simulink model "rev0BB"  (R2017b)
settings: Solver=FixedStepDiscrete  StartTime=0  StopTime=(((preLen+100+dataLenSymbols)*1+pad_first*3)*basePer)  RelTol=1e-3
values from neighbouring files (symbols this model uses):
  ack_stf_len_symbols = length(x_ACK_STF)    [rev0BB_setup.m]
  agc_delay_lag = 32    [rev0BB_setup.m]
  agc_detector_coef = ones(1,agc_detector_taps)./agc_detector_taps    [rev0BB_setup.m]
  agc_on = true    [rev0BB_startup.m]
  agc_sat_low = -agcSaturation    (= -12)    [rev0BB_setup.m]
  agc_sat_up = agcSaturation    (= 12)    [rev0BB_setup.m]
  agcDesired = 0    [rev0BB_setup.m]
  agcExpDomain = agcSaturation    (= 12)    [rev0BB_setup.m]
  agcExpResolution = 2^-5    (= 0.03125)    [rev0BB_setup.m]
  agcPwrAvgNum = 128    [rev0BB_setup.m]
  agcSaturation = 12    [rev0BB_setup.m]
  agcSettleThresh = 0.65    [rev0BB_setup.m]
  agcStep = 2^-8    (= 0.00390625)    [rev0BB_setup.m]
  atanDomain = 5    [rev0BB_setup.m]
  atanDomainTiming = 256    [rev0BB_setup.m]
  atanResolution = 2^-9    (= 0.001953125)    [rev0BB_setup.m]
  atanResolutionTiming = 2^-5    (= 0.03125)    [rev0BB_setup.m]
  averaging_num = ones(1, averaging_samples)    [rev0BB_setup.m]
  averaging_samples = 128    [rev0BB_setup.m]
  awgnSeed = abs(dBSnrRange(dBSnrInd)*1000+trial+10000000)    [plotBer.m]    (also in rev0BB_startup.m = 67)
  basePer = 1/baseFreq    (= 5e-08)    [rev0BB_setup.m]
  bitsPerSymbolHeader = log2(radixHeader)    [rev0BB_setup.m]
  bitsPerSymbolMax = log2(radixMax)    [rev0BB_setup.m]
  cal_sig_i_mult = 1.0    (= 1)    [rev0BB_startup.m]
  cal_sig_i_offset = 0.0    (= 0)    [rev0BB_startup.m]
  cal_sig_q_mult = 1.0    (= 1)    [rev0BB_startup.m]
  cal_sig_q_offset = 0.0    (= 0)    [rev0BB_startup.m]
  cefEarlyWarning = 256    [rev0BB_setup.m]
  cefLen = length(x_CEF)    [rev0BB_setup.m]
  channelFIR = zeros(1, round(maxSampleDelay)+1)    [rev0BB_startup.m]
  coarseCFOAdaptDelay = 1    [rev0BB_setup.m]
  cr_i = 0.020    (= 0.02)    [rev0BB_setup.m]
  cr_i_preamp = 2^-9    (= 0.001953125)    [rev0BB_setup.m]
  cr_int1_sat_low = -cr_integrator1_saturation    (= -0.6)    [rev0BB_setup.m]
  cr_int1_sat_up = cr_integrator1_saturation    (= 0.6)    [rev0BB_setup.m]
  cr_integrator1_decay = 1    [rev0BB_setup.m]
  cr_integrator1_saturation = 0.6    [rev0BB_setup.m]
  cr_mult_pipeline = 0    [rev0BB_setup.m]
  cr_p = 0.015    [rev0BB_setup.m]
  cr_sat2_low = -cr_saturation2    (= -0.6)    [rev0BB_setup.m]
  cr_sat2_up = cr_saturation2    (= 0.6)    [rev0BB_setup.m]
  cr_smooth_num = (1/cr_smooth_samples).*ones(1, cr_smooth_samples)    [rev0BB_setup.m]
  D_128 = [ 1,  8,  2,  4, 16, 32, 64]    [golay.m]    (also in rev0BB_setup.m)
  D_32 = [ 1,  4,  8,  2, 16]    [golay.m]    (also in rev0BB_setup.m)
  dataLenSymbols = header_len_bytes*8/bitsPerSymbolHeader + frame_len_bytes*8/bitsPerSymbol    [rev0BB_setup.m]
  default_channel = 3    [rev0BB_setup.m]
  dmm_coefs = ones(1,dmm_samples)./dmm_samples    [rev0BB_setup.m]
  dst_field_len = 8    [rev0BB_setup.m]
  expDomain = 3.3    [rev0BB_setup.m]
  expResolution = 2^-5    (= 0.03125)    [rev0BB_setup.m]
  expTol = .1    (= 0.1)    [rev0BB_setup.m]
  flush_delay = regular_pipeline*2+mult_pipeline+4    (= 4)    [rev0BB_setup.m]
  frac_lut_domain = 256    [rev0BB_setup.m]
  frac_lut_domain_cr = 64    [rev0BB_setup.m]
  frac_lut_range_max = 512    [rev0BB_setup.m]
  frac_lut_range_max_coarse_cfo = 127    [rev0BB_setup.m]
  frac_lut_range_max_cr = 127    [rev0BB_setup.m]
  frac_lut_range_min = -frac_lut_range_max    (= -512)    [rev0BB_setup.m]
  frac_lut_range_min_coarse_cfo = -frac_lut_range_max_coarse_cfo    (= -127)    [rev0BB_setup.m]
  frac_lut_range_min_cr = -frac_lut_range_max_cr    (= -127)    [rev0BB_setup.m]
  frac_lut_table_breaks = -frac_lut_domain:frac_lut_res:(frac_lut_domain-1)    [rev0BB_setup.m]
  frac_lut_table_breaks_coarse_cfo = -frac_lut_domain_coarse_cfo:frac_lut_res_coarse_cfo:(frac_lut_domain_coarse_cfo-1)    [rev0BB_setup.m]
  frac_lut_table_breaks_cr = -frac_lut_domain_cr:frac_lut_res_cr:(frac_lut_domain_cr-1)    [rev0BB_setup.m]
  frac_lut_table_data = 1./frac_lut_table_breaks    [rev0BB_setup.m]
  frac_lut_table_data_coarse_cfo = 1./frac_lut_table_breaks_coarse_cfo    [rev0BB_setup.m]
  frac_lut_table_data_cr = 1./frac_lut_table_breaks_cr    [rev0BB_setup.m]
  freeze_en_agc = true    [rev0BB_startup.m]
  freeze_en_cr_int1 = false    [rev0BB_startup.m]
  freeze_en_cr_int2 = false    [rev0BB_startup.m]
  freeze_en_cr_phase = false    [rev0BB_startup.m]
  freeze_en_tr_int1 = false    [rev0BB_startup.m]
  freeze_en_tr_int2 = false    [rev0BB_startup.m]
  freeze_en_tr_phase = false    [rev0BB_startup.m]
  freeze_on_cef_done = true    [rev0BB_startup.m]
  freeze_on_stf_done = false    [rev0BB_startup.m]
  freeze_on_valid = true    [rev0BB_startup.m]
  golay_type = 32    [rev0BB_setup.m]
  guardInt = int16(4)    [rev0BB_setup.m]
  guardTol = int16(5)    [rev0BB_setup.m]
  header_len_bytes = 8    [rev0BB_setup.m]
  lineWidth = 60    [rev0BB_setup.m]
  lmsEqDepth = 38    [rev0BB_setup.m]
  lmsStep_init = 0.006    [rev0BB_setup.m]
  lmsStep_meta = (lmsStep_final - lmsStep_init)/cefLen    [rev0BB_setup.m]
  lnDomain = 16    [rev0BB_setup.m]
  lnResolution = 2^-5    (= 0.03125)    [rev0BB_setup.m]
  local_node_id = 2    [rev0BB_startup.m]
  maxMsgSize = length(xSpectrum_PRE)+dataLenSymbols+300    [rev0BB_setup.m]
  minSTFPeaks = 3    [rev0BB_setup.m]
  mod_scheme_len_bytes = 1    [rev0BB_setup.m]
  modBPS = [1, 2, 4]    [rev0BB_setup.m]
  modKeys = [0, 1, 2]    [rev0BB_setup.m]
  mult_pipeline = 0    [rev0BB_setup.m]
  overSampleFreq = 80e6    (= 80000000)    [rev0BB_setup.m]
  overSamplePer = 1/overSampleFreq    (= 1.25e-08)    [rev0BB_setup.m]
  pad_first = 1000    [createTestVectors.m]
  post_cr_i_offset = 0    [rev0BB_startup.m]
  post_cr_q_offset = 0    [rev0BB_startup.m]
  preambleSequentialDetect = 2    [rev0BB_setup.m]
  preLen = length(x_PRE)    [rev0BB_setup.m]
  qam16_demod_scale_factor = qam16_hdl_distance/qam16_power_normalized_distance    [rev0BB_setup.m]
  rcRxFilt = [0.000303163120401141 -0.00118915940834234 -0.00187387637177 -0.00124167532697737 0.00029186889076529 0.00164526160586517 0.00182432050803312 0.000652133621739543 -0.00105668254004908 -0.00204011570659167 -0.00150058088768918 0.00026138356356816 0.0019831869994874 0.00231075800085521 0.000821993419120097 -0.00154687337975486 -0.00305430783933469 -0.00238186490079127 0.000301216962040692 0.00325307 ...(+2001 chars)    [rev0BB_setup.m]
  rcTxFilt = [0.000303163120401141 -0.00118915940834234 -0.00187387637177 -0.00124167532697737 0.00029186889076529 0.00164526160586517 0.00182432050803312 0.000652133621739543 -0.00105668254004908 -0.00204011570659167 -0.00150058088768918 0.00026138356356816 0.0019831869994874 0.00231075800085521 0.000821993419120097 -0.00154687337975486 -0.00305430783933469 -0.00238186490079127 0.000301216962040692 0.00325307 ...(+2001 chars)    [rev0BB_setup.m]
  regular_pipeline = 0    [rev0BB_setup.m]
  rx_gain = 1    [rev0BB_setup.m]
  rx_gain_i = 1    [rev0BB_setup.m]
  rx_gain_q = 1    [rev0BB_setup.m]
  rx_impare_i_offset = 0    [rev0BB_startup.m]
  rx_impare_i_scale = 1    [rev0BB_startup.m]
  rx_impare_q_offset = 0    [rev0BB_startup.m]
  rx_impare_q_scale = 1    [rev0BB_startup.m]
  rx_offset_correction_i = 0    [rev0BB_startup.m]
  rx_offset_correction_q = 0    [rev0BB_startup.m]
  sin_source_amp = 1    [rev0BB_setup.m]
  sin_source_freq = 250e6/16    (= 15625000)    [rev0BB_setup.m]
  slowPer = overSamplePer*slowSample    (= 2.5e-08)    [rev0BB_setup.m]
  std_pkt_type = 0    [rev0BB_setup.m]
  stfLen = length(x_STF)    [rev0BB_setup.m]
  testMsg = cat(1, xCTRL_PRE_adj, header, payload)    [plotBer.m]
  timing_i = 0.25    [rev0BB_setup.m]
  ... (+25 more)
undefined symbols (not defined in the file or in its folder): cr_integrator2_saturation, doppler, i, magnitude, useFadingChannel
libraries: helperLib x128, simulink x90, golayLib x34, dspsigops x32, commfilt2 x27, commdigbbndpm3 x8, hdlsllib x6, dsparch4 x4, commdigbbndam3 x4, commchan3 x2, commrflib2 x2, commcrc2 x2
(part 2 of 10)

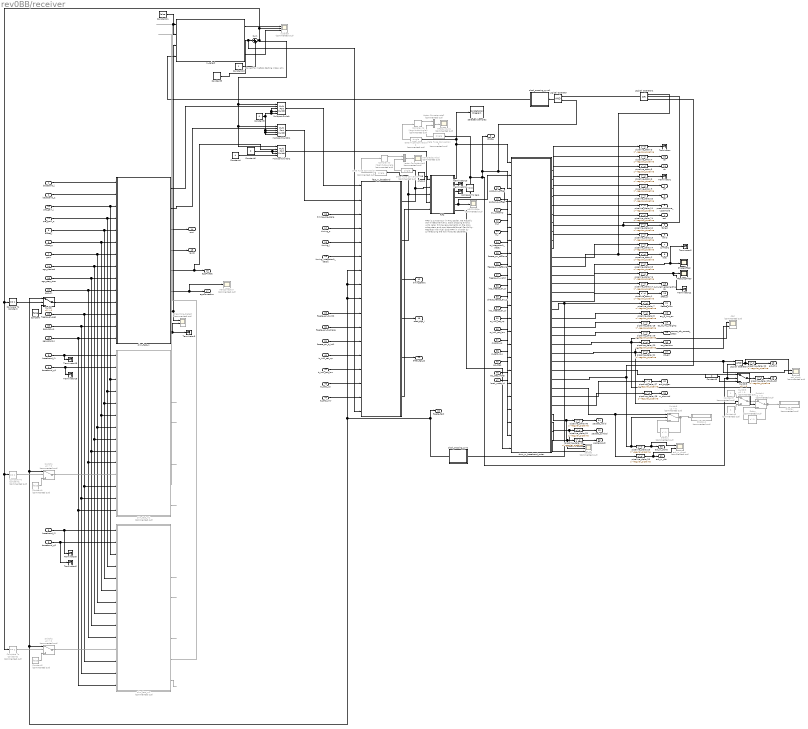
== system rev0BB/receiver ==
  note: Correct for matlab starting index at 1
  note: FIFO is syncronous in HDL Coder.
      | We actually don't need/want this.
      | Clock crossing allows us to relax timing
      | requirements on the slow subsystem
      | and provides additional flexibility.
      |
      | Replace with dual clock FIFO in Vivado
      | by synthesizing the two modules seperatly
  baseband_i : Inport  SampleTime=overSamplePer
  baseband_q : Inport  Port=2  SampleTime=overSamplePer
  baseband_i1 : Inport  Port=3  OutDataTypeStr=fixdt(1,14,10)  SampleTime=overSamplePer
  baseband_q1 : Inport  Port=4  OutDataTypeStr=fixdt(1,14,10)  SampleTime=overSamplePer
  baseband_i2 : Inport  Port=5  OutDataTypeStr=fixdt(1,14,10)  SampleTime=overSamplePer
  baseband_q2 : Inport  Port=6  OutDataTypeStr=fixdt(1,14,10)  SampleTime=overSamplePer
  gain : Inport  Port=7  SampleTime=overSamplePer
  offset_i : Inport  Port=8  SampleTime=overSamplePer
  offset_q : Inport  Port=9  SampleTime=overSamplePer
  pre_gain_i : Inport  Port=10  SampleTime=overSamplePer
  pre_gain_q : Inport  Port=11  SampleTime=overSamplePer
  post_cr_i_offset : Inport  Port=12
  post_cr_q_offset : Inport  Port=13
  agc_desired : Inport  Port=14
  agc_step_size : Inport  Port=15
  timing_pre_scale : Inport  Port=16
  timing_p : Inport  Port=17
  timing_i : Inport  Port=18
  timing_integrator1_decay : Inport  Port=19
  agc_on : Inport  Port=20  OutDataTypeStr=boolean
  cr_i_preamp : Inport  Port=21
  cr_p : Inport  Port=22
  cr_i : Inport  Port=23
  cr_integrator1_decay : Inport  Port=24
  freeze_on_stfDone : Inport  Port=25
  freeze_on_cefDone : Inport  Port=26
  freeze_on_valid : Inport  Port=27
  freeze_en_agc : Inport  Port=28
  freeze_en_tr_int2 : Inport  Port=29
  freeze_en_tr_phase : Inport  Port=30
  freeze_en_tr_int1 : Inport  Port=31
  int2_freeze_en_cr : Inport  Port=32  OutDataTypeStr=boolean
  phase_freeze_en_cr : Inport  Port=33  OutDataTypeStr=boolean
  int1_freeze_en_cr : Inport  Port=34  OutDataTypeStr=boolean
  cr_int1_sat_up : Inport  Port=35
  cr_int1_sat_low : Inport  Port=36
  cr_sat2_up : Inport  Port=37
  cr_sat2_low : Inport  Port=38
  agc_sat_up : Inport  Port=39
  agc_sat_low : Inport  Port=40
  tr_int1_sat_up : Inport  Port=41
  tr_int1_sat_low : Inport  Port=42
  tr_sat2_up : Inport  Port=43
  tr_sat2_low : Inport  Port=44
  eq_step : Inport  Port=45
  eq_step_meta : Inport  Port=46
  local_node_id : Inport  Port=47
  AGCCorrection : Scope  Commented=on
  AGCPWREst : Scope  Commented=on
  AfterLoopFilter : Scope
  Always : Constant  Value=true  OutDataTypeStr=boolean  SampleTime=-1
  CRC : Scope  Commented=on  NumInputPorts=2
  Compare To Constant : simulink/Logic and Bit Operations/Compare To Constant  relop===  const=1  OutDataTypeStr=boolean
  Compare To Constant1 : simulink/Logic and Bit Operations/Compare To Constant  Commented=on  relop===  const=2  OutDataTypeStr=boolean
  Compare To Constant2 : simulink/Logic and Bit Operations/Compare To Constant  Commented=on  relop===  const=3  OutDataTypeStr=boolean
  Compare To Zero : simulink/Logic and Bit Operations/Compare To Zero  relop=<=  OutDataTypeStr=boolean
  Complex to Magnitude-Angle : ComplexToMagnitudeAngle  Commented=on
  Complex to Magnitude-Angle1 : ComplexToMagnitudeAngle  Commented=on
  Constant : Constant  Value=false  OutDataTypeStr=Inherit: Inherit via back propagation  SampleTime=-1
  Constant1 : Constant  Commented=on  Value=false  OutDataTypeStr=Inherit: Inherit via back propagation  SampleTime=-1
  Constant10 : Constant  OutDataTypeStr=uint8  SampleTime=-1
  Constant11 : Constant  Value=false  OutDataTypeStr=boolean  SampleTime=-1
  Constant2 : Constant  Commented=on  Value=false  OutDataTypeStr=Inherit: Inherit via back propagation  SampleTime=-1
  Constant3 : Constant  Value=0  OutDataTypeStr=single  SampleTime=-1
  Constant4 : Constant  Value=4  OutDataTypeStr=single  SampleTime=-1
  Constant5 : Constant  Value=uint8(0)  SampleTime=-1
  Constant6 : Constant  Value=0  OutDataTypeStr=single  SampleTime=-1
  Constant7 : Constant  Commented=on
  Constant8 : Constant  Commented=on  Value=2
  Constant9 : Constant  Value=0  OutDataTypeStr=Inherit: Inherit via back propagation  SampleTime=-1
  Data Type Conversion{,1..3} (4 alike) : DataTypeConversion  Commented=on  OutDataTypeStr=single
  Delay : Delay  Commented=on  DelayLength=1  InitialCondition=0
  Delay1 : Delay  Commented=on  DelayLength=1  InitialCondition=0
  Display : Display  Commented=on
  Display1 : Display  Commented=on
  FIFO : Subsystem
  FIFOSymbols : Scope  Commented=on
  Logical Operator : Logic  AllPortsSameDT=off  OutDataTypeStr=boolean
  Logical Operator1 : Logic  Operator=OR  Inputs=3  AllPortsSameDT=off  OutDataTypeStr=boolean
  Logical Operator3 : Logic  AllPortsSameDT=off  OutDataTypeStr=boolean
  Multiport Switch : MultiPortSwitch  Inputs=4
  Multiport Switch1 : MultiPortSwitch  Inputs=4
  Multiport Switch2 : MultiPortSwitch  Inputs=4
  PhaseOffset : Scope
  Preamble_Detect : Scope  Commented=on  NumInputPorts=2
  SampledSymbol : Scope  Commented=on
  Selected Samples : ConstellationDiagram
  Sum : Sum  Inputs=|++
  Switch : Switch  Criteria=u2 > Threshold
  Switch{1..4,6} (5 alike) : Switch  Commented=on  Criteria=u2 > Threshold
  Switch5 : Switch  Criteria=u2 > Threshold
  Terminator{,1..3,5..6,12..16} (11 alike) : Terminator
  Vector Concatenate2 : Concatenate  Commented=on  Mode=Multidimensional array  ConcatenateDimension=2
  Vector Concatenate3 : Concatenate  Commented=on  Mode=Multidimensional array  ConcatenateDimension=2
  ack_check : Scope  Commented=on  NumInputPorts=2
  ack_rx_check : Scope  Commented=on  NumInputPorts=2
  clock_crossing_sync : Subsystem
  clock_crossing_sync1 : Subsystem
  fast_rx_baseband : Subsystem  TreatAsAtomicUnit=on
  packed : Scope  Commented=on  NumInputPorts=4
  pipeline_delay{1..31} (31 alike) : Delay  DelayLength=regular_pipeline
  rxSelect : Scope  Commented=on  NumInputPorts=3
  rx_select : Subsystem  TreatAsAtomicUnit=on
  slim_fast_rx : Subsystem  TreatAsAtomicUnit=on
  slim_fast_rx1 : Subsystem  Commented=on
  slim_fast_rx2 : Subsystem  Commented=on
  slow_rx_baseband_outer : Subsystem  TreatAsAtomicUnit=on
  stf : Outport
  cef : Outport  Port=2
  preambleDone_upsample : Outport  Port=3
  ack : Outport  Port=4
  failed : Outport  Port=5
  valid : Outport  Port=6
  symbols : Outport  Port=7
  last : Outport  Port=8
  strobe : Outport  Port=9
  ca : Outport  Port=10
  cb : Outport  Port=11
  timingDelay : Outport  Port=12
  cumulativeCarrierPhase : Outport  Port=13
  rawI : Outport  Port=14
  rawQ : Outport  Port=15
  agcPwrEst : Outport  Port=16
  agcCorrection : Outport  Port=17
  after_cr : Outport  Port=18
  after_agc_I : Outport  Port=19
  after_agc_Q : Outport  Port=20
  freeze_slow : Outport  Port=21
  freeze_fast : Outport  Port=22
  eq_ff_lms_err : Outport  Port=23
  eq_ff_lms_weights : Outport  Port=24  SampleTime=slowPer
  coarse_cfo_correct_steps : Outport  Port=25  SampleTime=slowPer
  crc_decision : Outport  Port=26  SampleTime=slowPer
  crc_err : Outport  Port=27  SampleTime=slowPer
  ack_this : Outport  Port=28  SampleTime=slowPer
  ack_dst : Outport  Port=29  SampleTime=slowPer
  ack_rx_done : Outport  Port=30  SampleTime=slowPer
  ack_rx_dst : Outport  Port=31  SampleTime=slowPer
  ack_trigger : Outport  Port=32  SampleTime=slowPer
  rx_channel : Outport  Port=33  SampleTime=slowPer
  packed_valid : Outport  Port=34
  packed_symbol : Outport  Port=35
  packed_last : Outport  Port=36  SampleTime=slowPer
  wires:
  pipeline_delay4/1 -> ca/1
  pipeline_delay5/1 -> cb/1
  pipeline_delay9/1 -> stf/1
  pipeline_delay10/1 -> cef/1
  pipeline_delay11/1 -> preambleDone_upsample/1
  pipeline_delay12/1 -> failed/1
  pipeline_delay13/1 -> valid/1
  pipeline_delay14/1 -> symbols/1
  pipeline_delay15/1 -> Terminator2/1, PhaseOffset/1
  pipeline_delay16/1 -> Terminator12/1, AfterLoopFilter/1
  pipeline_delay17/1 -> cumulativeCarrierPhase/1
  FIFO/4(empty) -> Compare To Zero/1
  Compare To Zero/1 -> Data Type Conversion3/1, strobe/1, Logical Operator/2, slow_rx_baseband_outer/3(enb), Switch5/2, Logical Operator3/2
  pre_gain_i/1 -> slim_fast_rx2/3(pre_gain_i), slim_fast_rx1/3(pre_gain_i), slim_fast_rx/3(pre_gain_i)
  pre_gain_q/1 -> slim_fast_rx2/4(pre_gain_q), slim_fast_rx1/4(pre_gain_q), slim_fast_rx/4(pre_gain_q)
  offset_i/1 -> slim_fast_rx2/5(offset_i), slim_fast_rx1/5(offset_i), slim_fast_rx/5(offset_i)
  offset_q/1 -> slim_fast_rx2/6(offset_q), slim_fast_rx1/6(offset_q), slim_fast_rx/6(offset_q)
  baseband_i/1 -> slim_fast_rx/1(baseband_i)
  baseband_q/1 -> slim_fast_rx/2(baseband_q)
  gain/1 -> slim_fast_rx2/7(gain), slim_fast_rx1/7(gain), slim_fast_rx/7(gain)
  fast_rx_baseband/3(timing_delay) -> timingDelay/1
  slim_fast_rx/3(rawI) -> rawI/1
  slim_fast_rx/4(rawQ) -> rawQ/1
  Vector Concatenate3/1 -> SampledSymbol/1
  Complex to Magnitude-Angle/1 -> Vector Concatenate3/1
  Data Type Conversion/1 -> Vector Concatenate3/2
  Data Type Conversion1/1 -> Complex to Magnitude-Angle/1
  Complex to Magnitude-Angle1/1 -> Vector Concatenate2/1
  Vector Concatenate2/1 -> FIFOSymbols/1
  Data Type Conversion2/1 -> Complex to Magnitude-Angle1/1
  Data Type Conversion3/1 -> Vector Concatenate2/2
  slim_fast_rx/5(agcPwrEst) -> Multiport Switch2/2, agcPwrEst/1
  slow_rx_baseband_outer/2(ca) -> pipeline_delay4/1
  slow_rx_baseband_outer/3(cb) -> pipeline_delay5/1
  slow_rx_baseband_outer/5(stf) -> pipeline_delay9/1
  slow_rx_baseband_outer/6(cef) -> pipeline_delay10/1
  slow_rx_baseband_outer/7(preamble_done) -> pipeline_delay11/1
  slow_rx_baseband_outer/9(failed) -> Logical Operator1/2, pipeline_delay12/1
  slow_rx_baseband_outer/10(valid) -> pipeline_delay13/1
  slow_rx_baseband_outer/11(symbols) -> pipeline_delay14/1
  slow_rx_baseband_outer/13(carrier_phase_offset) -> pipeline_delay15/1
  slow_rx_baseband_outer/14(carrier_phase_filtered) -> pipeline_delay16/1
  slow_rx_baseband_outer/15(carrier_phase_correction) -> pipeline_delay17/1
  fast_rx_baseband/1(push) -> Data Type Conversion/1, FIFO/2(push)
  Always/1 -> FIFO/1(pop)
  slow_rx_baseband_outer/16(after_cr) -> pipeline_delay1/1
  pipeline_delay1/1 -> after_cr/1
  fast_rx_baseband/4(after_agc_I) -> after_agc_I/1
  fast_rx_baseband/5(after_agc_Q) -> after_agc_Q/1
  post_cr_i_offset/1 -> slow_rx_baseband_outer/4(post_cr_i_offset)
  post_cr_q_offset/1 -> slow_rx_baseband_outer/5(post_cr_q_offset)
  agc_step_size/1 -> slim_fast_rx2/9(agc_step_size), slim_fast_rx1/9(agc_step_size), slim_fast_rx/9(agc_step_size)
  agc_desired/1 -> slim_fast_rx2/8(agc_desired), slim_fast_rx1/8(agc_desired), slim_fast_rx/8(agc_desired)
  timing_pre_scale/1 -> fast_rx_baseband/3(timing_pre_scale)
  timing_p/1 -> fast_rx_baseband/4(timing_p)
  timing_i/1 -> fast_rx_baseband/5(timing_i)
  timing_integrator1_decay/1 -> fast_rx_baseband/6(timing_integrator1_decay)
  cr_i_preamp/1 -> slow_rx_baseband_outer/6(cr_i_preamp)
  cr_p/1 -> slow_rx_baseband_outer/7(cr_p)
  cr_i/1 -> slow_rx_baseband_outer/8(cr_i)
  cr_integrator1_decay/1 -> slow_rx_baseband_outer/9(cr_integrator1_decay)
  agc_on/1 -> slim_fast_rx2/10(agc_on), slim_fast_rx1/10(agc_on), slim_fast_rx/10(agc_on)
  freeze_on_stfDone/1 -> slow_rx_baseband_outer/10(freeze_on_stfDone)
  freeze_on_cefDone/1 -> slow_rx_baseband_outer/11(freeze_on_cefDone)
  freeze_on_valid/1 -> slow_rx_baseband_outer/12(freeze_on_valid)
  slow_rx_baseband_outer/17(freeze) -> clock_crossing_sync/1(In1), pipeline_delay7/1
  clock_crossing_sync/1(Out1) -> Switch2/1, Switch1/1, Switch/1, fast_rx_baseband/7(tr_int2_freeze), fast_rx_baseband/8(tr_phase_freeze), fast_rx_baseband/9(tr_int1_freeze), freeze_fast/1
  int2_freeze_en_cr/1 -> slow_rx_baseband_outer/13(int2_freeze_en_cr)
  freeze_en_agc/1 -> slim_fast_rx2/12(freeze_en_agc), slim_fast_rx1/12(freeze_en_agc), slim_fast_rx/12(freeze_en_agc)
  freeze_en_tr_int2/1 -> fast_rx_baseband/10(freeze_en_tr_int2)
  freeze_en_tr_phase/1 -> fast_rx_baseband/11(freeze_en_tr_phase)
  cr_int1_sat_up/1 -> slow_rx_baseband_outer/16(cr_int1_sat_up)
  cr_int1_sat_low/1 -> slow_rx_baseband_outer/17(cr_int1_sat_low)
  cr_sat2_up/1 -> slow_rx_baseband_outer/18(cr_sat2_up)
  cr_sat2_low/1 -> slow_rx_baseband_outer/19(cr_sat2_low)
  agc_sat_up/1 -> slim_fast_rx2/13(agc_sat_up), slim_fast_rx1/13(agc_sat_up), slim_fast_rx/13(agc_sat_up)
  agc_sat_low/1 -> slim_fast_rx2/14(agc_sat_low), slim_fast_rx1/14(agc_sat_low), slim_fast_rx/14(agc_sat_low)
  tr_int1_sat_up/1 -> fast_rx_baseband/13(tr_int1_sat_up)
  tr_int1_sat_low/1 -> fast_rx_baseband/14(tr_int1_sat_low)
  phase_freeze_en_cr/1 -> slow_rx_baseband_outer/14(phase_freeze_en_cr)
  int1_freeze_en_cr/1 -> slow_rx_baseband_outer/15(int1_freeze_en_cr)
  freeze_en_tr_int1/1 -> fast_rx_baseband/12(freeze_en_tr_int1)
  tr_sat2_low/1 -> fast_rx_baseband/16(tr_sat2_low)
  tr_sat2_up/1 -> fast_rx_baseband/15(tr_sat2_up)
  slow_rx_baseband_outer/12(last) -> Logical Operator1/1, pipeline_delay2/1
  slim_fast_rx/6(agcCorrection) -> AGCCorrection/1, agcCorrection/1
  slow_rx_baseband_outer/18(eq_ff_lms_err) -> pipeline_delay8/1
  FIFO/5(agc_out) -> slow_rx_baseband_outer/2(agc_pwr_est), AGCPWREst/1
  fast_rx_baseband/2(data_out) -> Data Type Conversion1/1, FIFO/3(in)
  FIFO/1(out) -> slow_rx_baseband_outer/1(Data_In), Selected Samples/1, Data Type Conversion2/1
  eq_step/1 -> slow_rx_baseband_outer/20(eq_step)
  eq_step_meta/1 -> slow_rx_baseband_outer/21(eq_step_meta)
  slow_rx_baseband_outer/1(ca_pos) -> pipeline_delay3/1
  slow_rx_baseband_outer/4(cb_pos) -> pipeline_delay6/1
  pipeline_delay3/1 -> Terminator/1
  pipeline_delay6/1 -> Terminator1/1
  pipeline_delay7/1 -> freeze_slow/1
  pipeline_delay8/1 -> eq_ff_lms_err/1
  slow_rx_baseband_outer/19(eq_ff_lms_weights) -> pipeline_delay18/1
  slow_rx_baseband_outer/20(coarse_cfo_correct_steps) -> pipeline_delay19/1
  pipeline_delay18/1 -> eq_ff_lms_weights/1
  pipeline_delay19/1 -> coarse_cfo_correct_steps/1
  slim_fast_rx/7(preamble_detected) -> rx_select/3(preamble_detect1), Preamble_Detect/1
  slim_fast_rx/8(preamble_err) -> Terminator3/1, Preamble_Detect/2
  Switch/1 -> slim_fast_rx/11(agc_freeze)
  Switch2/1 -> slim_fast_rx2/11(agc_freeze)
  slim_fast_rx1/3(rawI) -> ?
  slim_fast_rx1/4(rawQ) -> ?
  slim_fast_rx1/8(preamble_err) -> ?
  slim_fast_rx1/6(agcCorrection) -> ?
  slim_fast_rx2/3(rawI) -> ?
  slim_fast_rx2/4(rawQ) -> ?
  slim_fast_rx2/8(preamble_err) -> ?
  slim_fast_rx2/6(agcCorrection) -> ?
  baseband_i1/1 -> Terminator15/1, slim_fast_rx1/1(baseband_i)
  baseband_q1/1 -> Terminator16/1, slim_fast_rx1/2(baseband_q)
  baseband_i2/1 -> Terminator5/1, slim_fast_rx2/1(baseband_i)
  baseband_q2/1 -> Terminator6/1, slim_fast_rx2/2(baseband_q)
  Compare To Constant/1 -> Switch/2
  pipeline_delay2/1 -> last/1
  Constant/1 -> Switch/3
  Constant1/1 -> Switch1/3
  Compare To Constant1/1 -> Switch1/2
  Switch1/1 -> slim_fast_rx1/11(agc_freeze)
  Constant2/1 -> Switch2/3
  Compare To Constant2/1 -> Switch2/2
  Logical Operator/1 -> clock_crossing_sync1/1(In1)
  Logical Operator1/1 -> Logical Operator/1
  Constant4/1 -> Multiport Switch2/5
  Sum/1 -> Multiport Switch/1, Multiport Switch2/1, Multiport Switch1/1, Compare To Constant2/1, Compare To Constant1/1, Compare To Constant/1, rxSelect/2
  clock_crossing_sync1/1(Out1) -> rx_select/4(pkt_done)
  slim_fast_rx1/7(preamble_detected) -> ?
  slim_fast_rx2/7(preamble_detected) -> ?
  rx_select/1(receiving) -> rxSelect/1
  rx_select/3(err) -> rxSelect/3
  Constant3/1 -> Multiport Switch/3, Multiport Switch/4, Multiport Switch/5, Multiport Switch1/3, Multiport Switch1/4, Multiport Switch1/5
  Constant6/1 -> Multiport Switch2/4, Multiport Switch2/3
  slim_fast_rx/1(sig_out_i) -> Multiport Switch/2
  slim_fast_rx/2(sig_out_q) -> Multiport Switch1/2
  slow_rx_baseband_outer/22(crc_err) -> CRC/2, pipeline_delay21/1, Switch3/2
  Switch3/1 -> Switch4/1
  Constant7/1 -> Switch3/1
  Constant8/1 -> Switch3/3
  Switch4/1 -> Display/1, Delay/1
  Delay/1 -> Switch4/3
  slow_rx_baseband_outer/21(crc_decision) -> CRC/1, pipeline_delay20/1, Switch4/2
  pipeline_delay20/1 -> crc_decision/1
  pipeline_delay21/1 -> crc_err/1
  pipeline_delay22/1 -> ack_this/1
  Switch5/1 -> pipeline_delay23/1
  local_node_id/1 -> slow_rx_baseband_outer/22(local_node_id)
  Logical Operator3/1 -> ack_check/2, pipeline_delay22/1
  slow_rx_baseband_outer/23(ack_this) -> ack_check/1, Logical Operator3/1
  slow_rx_baseband_outer/24(ack_dst) -> Switch5/1
  Constant9/1 -> Switch5/3
  pipeline_delay23/1 -> ack_dst/1
  pipeline_delay24/1 -> ack/1
  slow_rx_baseband_outer/8(ack) -> pipeline_delay24/1
  slow_rx_baseband_outer/25(ack_rx_done) -> Switch6/2, pipeline_delay25/1, Logical Operator1/3
  pipeline_delay26/1 -> ack_rx_check/2, ack_rx_dst/1
  Switch6/1 -> Display1/1, Delay1/1
  Delay1/1 -> Switch6/3
  slow_rx_baseband_outer/26(ack_rx_dst) -> Switch6/1, pipeline_delay26/1
  pipeline_delay25/1 -> ack_rx_check/1, ack_rx_done/1
  pipeline_delay27/1 -> ack_trigger/1
  slow_rx_baseband_outer/27(ack_trigger) -> pipeline_delay27/1
  Multiport Switch/1 -> fast_rx_baseband/1(sig_in_i)
  Multiport Switch1/1 -> fast_rx_baseband/2(sig_in_q)
  Multiport Switch2/1 -> FIFO/4(agc_in)
  Constant5/1 -> fast_rx_baseband/17(channel_in), Sum/1
  Constant10/1 -> Sum/2
  fast_rx_baseband/6(channel_out) -> FIFO/5(channel_in)
  FIFO/6(channel_out) -> slow_rx_baseband_outer/23(channel_in)
  pipeline_delay28/1 -> rx_channel/1
  slow_rx_baseband_outer/28(channel_out) -> pipeline_delay28/1
  Constant11/1 -> rx_select/2(preamble_detect2), rx_select/1(preamble_detect3)
  slow_rx_baseband_outer/30(packed_symbol) -> pipeline_delay31/1, packed/1
  slow_rx_baseband_outer/29(packed_valid) -> pipeline_delay30/1, packed/2
  slow_rx_baseband_outer/31(packed_last) -> pipeline_delay29/1, packed/3
  pipeline_delay29/1 -> packed_last/1
  pipeline_delay31/1 -> packed_symbol/1
  pipeline_delay30/1 -> packed_valid/1
  slow_rx_baseband_outer/32(packed_err) -> packed/4
  FIFO/2(full) -> Terminator13/1
  FIFO/3(num) -> Terminator14/1

== system rev0BB/transmitter ==
  symbol : Inport
  gain : Inport  Port=2
  zero : Inport  Port=3
  ModMode : Inport  Port=4
  transmitter_internal : Subsystem
  baseband_i : Outport
  baseband_q : Outport  Port=2
  wires:
  gain/1 -> transmitter_internal/2(gain)
  transmitter_internal/1(baseband_i) -> baseband_i/1
  transmitter_internal/2(baseband_q) -> baseband_q/1
  zero/1 -> transmitter_internal/3(zero)
  symbol/1 -> transmitter_internal/1(symbol)
  ModMode/1 -> transmitter_internal/4(ModMode)

== system rev0BB/receiver/FIFO ==
  pop : Inport
  push : Inport  Port=2
  in : Inport  Port=3
  agc_in : Inport  Port=4
  channel_in : Inport  Port=5
  HDL FIFO : hdlsllib/HDL RAMs/HDL FIFO  fifo_size=16  ratio=slowSample  push_msg=Ignore  pop_msg=Ignore  show_empty=on  show_full=on  show_num=on
      settings: SourceProductName=HDL Coder  SourceProductBaseCode=HD
  HDL FIFO1 : hdlsllib/HDL RAMs/HDL FIFO  fifo_size=16  ratio=slowSample  push_msg=Ignore  pop_msg=Ignore  show_empty=off  show_full=off  show_num=off
      settings: SourceProductName=HDL Coder  SourceProductBaseCode=HD
  HDL FIFO2 : hdlsllib/HDL RAMs/HDL FIFO  fifo_size=16  ratio=slowSample  push_msg=Ignore  pop_msg=Ignore  show_empty=off  show_full=off  show_num=off
      settings: SourceProductName=HDL Coder  SourceProductBaseCode=HD
  Rate Transition : RateTransition  InitialCondition=1  OutPortSampleTime=slowPer
  out : Outport  SampleTime=slowPer
  full : Outport  Port=2
  num : Outport  Port=3
  empty : Outport  Port=4
  agc_out : Outport  Port=5  SampleTime=slowPer
  channel_out : Outport  Port=6  SampleTime=slowPer
  wires:
  HDL FIFO/2 -> Rate Transition/1
  HDL FIFO/1 -> out/1
  push/1 -> HDL FIFO/2, HDL FIFO2/2, HDL FIFO1/2
  in/1 -> HDL FIFO/1
  pop/1 -> HDL FIFO/3, HDL FIFO2/3, HDL FIFO1/3
  HDL FIFO/4 -> num/1
  HDL FIFO/3 -> full/1
  Rate Transition/1 -> empty/1
  agc_in/1 -> HDL FIFO1/1
  HDL FIFO1/1 -> agc_out/1
  channel_in/1 -> HDL FIFO2/1
  HDL FIFO2/1 -> channel_out/1

== system rev0BB/receiver/clock_crossing_sync ==
  In1 : Inport
  Delay : Delay  DelayLength=1  InitialCondition=0
  Delay1 : Delay  DelayLength=1  InitialCondition=0
  Delay2 : Delay  DelayLength=1  InitialCondition=0
  Rate Transition : RateTransition
  Out1 : Outport
  wires:
  Delay/1 -> Rate Transition/1
  Rate Transition/1 -> Delay1/1
  Delay2/1 -> Out1/1
  In1/1 -> Delay/1
  Delay1/1 -> Delay2/1

== system rev0BB/receiver/clock_crossing_sync1 ==
  In1 : Inport
  Delay : Delay  DelayLength=1  InitialCondition=0
  Delay1 : Delay  DelayLength=1  InitialCondition=0
  Delay2 : Delay  DelayLength=1  InitialCondition=0
  Rate Transition : RateTransition
  Out1 : Outport
  wires:
  Delay/1 -> Rate Transition/1
  Rate Transition/1 -> Delay1/1
  Delay2/1 -> Out1/1
  In1/1 -> Delay/1
  Delay1/1 -> Delay2/1

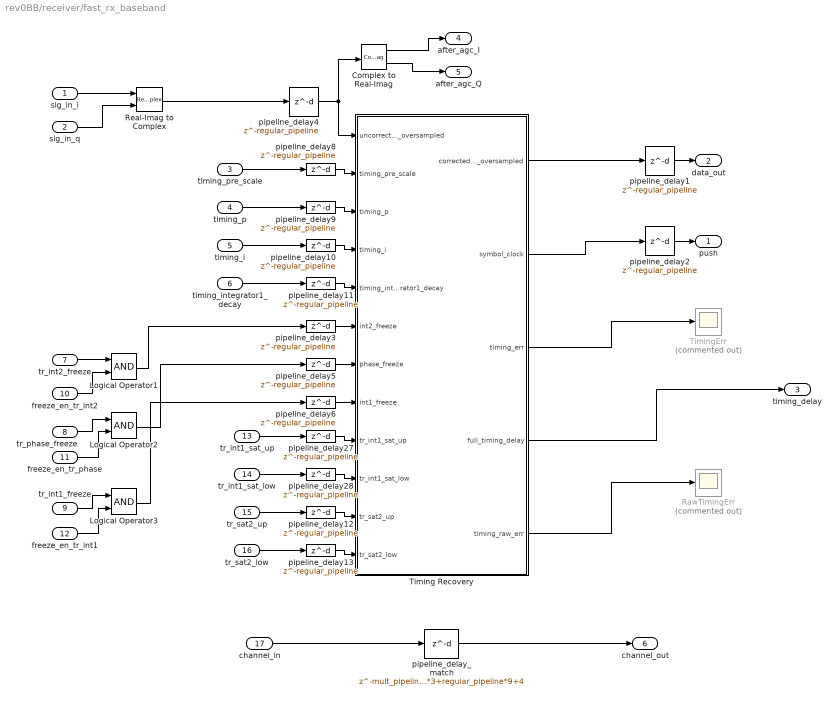
== system rev0BB/receiver/fast_rx_baseband ==
  sig_in_i : Inport
  sig_in_q : Inport  Port=2
  timing_pre_scale : Inport  Port=3
  timing_p : Inport  Port=4
  timing_i : Inport  Port=5
  timing_integrator1_decay : Inport  Port=6
  tr_int2_freeze : Inport  Port=7  OutDataTypeStr=boolean
  tr_phase_freeze : Inport  Port=8  OutDataTypeStr=boolean
  tr_int1_freeze : Inport  Port=9  OutDataTypeStr=boolean
  freeze_en_tr_int2 : Inport  Port=10  OutDataTypeStr=boolean
  freeze_en_tr_phase : Inport  Port=11  OutDataTypeStr=boolean
  freeze_en_tr_int1 : Inport  Port=12  OutDataTypeStr=boolean
  tr_int1_sat_up : Inport  Port=13
  tr_int1_sat_low : Inport  Port=14
  tr_sat2_up : Inport  Port=15
  tr_sat2_low : Inport  Port=16
  channel_in : Inport  Port=17
  Complex to Real-Imag : ComplexToRealImag
  Logical Operator1 : Logic  AllPortsSameDT=off  OutDataTypeStr=boolean
  Logical Operator2 : Logic  AllPortsSameDT=off  OutDataTypeStr=boolean
  Logical Operator3 : Logic  AllPortsSameDT=off  OutDataTypeStr=boolean
  RawTimingErr : Scope  Commented=on
  Real-Imag to Complex : RealImagToComplex
  Timing Recovery : Subsystem
  TimingErr : Scope  Commented=on
  pipeline_delay{1..6,8..13,27..28} (14 alike) : Delay  DelayLength=regular_pipeline
  pipeline_delay_match : Delay  DelayLength=mult_pipeline*3+regular_pipeline*9+4
  push : Outport
  data_out : Outport  Port=2
  timing_delay : Outport  Port=3
  after_agc_I : Outport  Port=4
  after_agc_Q : Outport  Port=5
  channel_out : Outport  Port=6
  wires:
  Timing Recovery/3(timing_err) -> TimingErr/1
  Timing Recovery/4(full_timing_delay) -> timing_delay/1
  Timing Recovery/5(timing_raw_err) -> RawTimingErr/1
  Timing Recovery/1(corrected_oversampled) -> pipeline_delay1/1
  Timing Recovery/2(symbol_clock) -> pipeline_delay2/1
  pipeline_delay1/1 -> data_out/1
  pipeline_delay2/1 -> push/1
  Complex to Real-Imag/1 -> after_agc_I/1
  Complex to Real-Imag/2 -> after_agc_Q/1
  pipeline_delay4/1 -> Timing Recovery/1(uncorrected_oversampled), Complex to Real-Imag/1
  timing_pre_scale/1 -> pipeline_delay8/1
  timing_p/1 -> pipeline_delay9/1
  timing_i/1 -> pipeline_delay10/1
  timing_integrator1_decay/1 -> pipeline_delay11/1
  pipeline_delay8/1 -> Timing Recovery/2(timing_pre_scale)
  pipeline_delay9/1 -> Timing Recovery/3(timing_p)
  pipeline_delay10/1 -> Timing Recovery/4(timing_i)
  pipeline_delay11/1 -> Timing Recovery/5(timing_integrator1_decay)
  tr_int2_freeze/1 -> Logical Operator1/1
  freeze_en_tr_int2/1 -> Logical Operator1/2
  Logical Operator1/1 -> pipeline_delay3/1
  tr_phase_freeze/1 -> Logical Operator2/1
  freeze_en_tr_phase/1 -> Logical Operator2/2
  Logical Operator2/1 -> pipeline_delay5/1
  pipeline_delay27/1 -> Timing Recovery/9(tr_int1_sat_up)
  pipeline_delay28/1 -> Timing Recovery/10(tr_int1_sat_low)
  tr_int1_sat_up/1 -> pipeline_delay27/1
  tr_int1_sat_low/1 -> pipeline_delay28/1
  tr_int1_freeze/1 -> Logical Operator3/1
  freeze_en_tr_int1/1 -> Logical Operator3/2
  Logical Operator3/1 -> pipeline_delay6/1
  tr_sat2_up/1 -> pipeline_delay12/1
  tr_sat2_low/1 -> pipeline_delay13/1
  pipeline_delay12/1 -> Timing Recovery/11(tr_sat2_up)
  pipeline_delay13/1 -> Timing Recovery/12(tr_sat2_low)
  Real-Imag to Complex/1 -> pipeline_delay4/1
  sig_in_i/1 -> Real-Imag to Complex/1
  sig_in_q/1 -> Real-Imag to Complex/2
  pipeline_delay3/1 -> Timing Recovery/6(int2_freeze)
  pipeline_delay5/1 -> Timing Recovery/7(phase_freeze)
  pipeline_delay6/1 -> Timing Recovery/8(int1_freeze)
  channel_in/1 -> pipeline_delay_match/1
  pipeline_delay_match/1 -> channel_out/1

== system rev0BB/receiver/rx_select ==
  preamble_detect3 : Inport
  preamble_detect2 : Inport  Port=2
  preamble_detect1 : Inport  Port=3
  pkt_done : Inport  Port=4
  Delay{,1..6} (7 alike) : Delay  DelayLength=1  InitialCondition=0
  rx_select : Stateflow chart  TreatAsAtomicUnit=on
  receiving : Outport
  select : Outport  Port=2
  err : Outport  Port=3
  wires:
  rx_select/2(select) -> Delay5/1
  preamble_detect2/1 -> Delay1/1
  preamble_detect3/1 -> Delay/1
  rx_select/1(receiving) -> Delay4/1
  rx_select/3(err) -> Delay6/1
  pkt_done/1 -> Delay3/1
  preamble_detect1/1 -> Delay2/1
  Delay/1 -> rx_select/1(preamble_detect3)
  Delay1/1 -> rx_select/2(preamble_detect2)
  Delay2/1 -> rx_select/3(preamble_detect1)
  Delay3/1 -> rx_select/4(done)
  Delay4/1 -> receiving/1
  Delay5/1 -> select/1
  Delay6/1 -> err/1

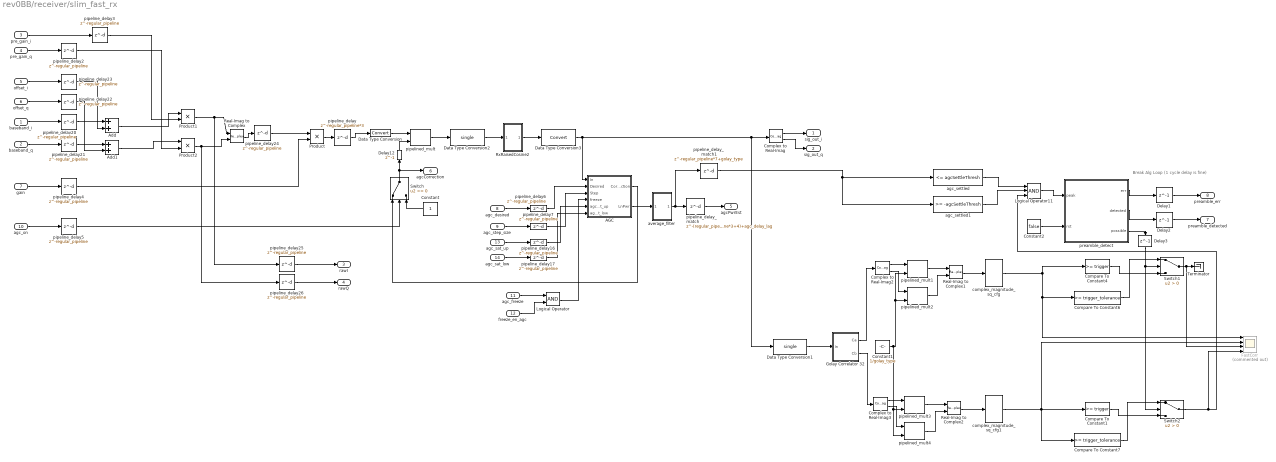
== system rev0BB/receiver/slim_fast_rx ==
  note: Break Alg Loop (1 cycle delay is fine)
  baseband_i : Inport
  baseband_q : Inport  Port=2
  pre_gain_i : Inport  Port=3
  pre_gain_q : Inport  Port=4
  offset_i : Inport  Port=5
  offset_q : Inport  Port=6
  gain : Inport  Port=7
  agc_desired : Inport  Port=8
  agc_step_size : Inport  Port=9
  agc_on : Inport  Port=10  OutDataTypeStr=boolean
  agc_freeze : Inport  Port=11  OutDataTypeStr=boolean
  freeze_en_agc : Inport  Port=12  OutDataTypeStr=boolean
  agc_sat_up : Inport  Port=13
  agc_sat_low : Inport  Port=14
  AGC : Subsystem  TreatAsAtomicUnit=on
  Add : Sum
  Add1 : Sum
  Compare To Constant1 : simulink/Logic and Bit Operations/Compare To Constant  relop=>=  const=trigger  OutDataTypeStr=boolean
  Compare To Constant4 : simulink/Logic and Bit Operations/Compare To Constant  relop=>=  const=trigger  OutDataTypeStr=boolean
  Compare To Constant6 : simulink/Logic and Bit Operations/Compare To Constant  relop=>=  const=trigger_tolerance  OutDataTypeStr=boolean
  Compare To Constant7 : simulink/Logic and Bit Operations/Compare To Constant  relop=>=  const=trigger_tolerance  OutDataTypeStr=boolean
  Complex to Real-Imag : ComplexToRealImag
  Complex to Real-Imag2 : ComplexToRealImag
  Complex to Real-Imag3 : ComplexToRealImag
  Constant : Constant  OutDataTypeStr=Inherit: Inherit via back propagation  SampleTime=-1
  Constant1 : Constant  Value=1/golay_type  OutDataTypeStr=Inherit: Inherit via back propagation  SampleTime=-1
  Constant2 : Constant  Value=false  SampleTime=-1
  Data Type Conversion : DataTypeConversion
  Data Type Conversion1 : DataTypeConversion  OutDataTypeStr=single
  Data Type Conversion2 : DataTypeConversion  OutDataTypeStr=single
  Data Type Conversion3 : DataTypeConversion
  Delay1 : Delay  DelayLength=1  InitialCondition=0
  Delay12 : Delay  DelayLength=1
  Delay2 : Delay  DelayLength=1  InitialCondition=0
  Delay3 : Delay  DelayLength=1  InitialCondition=0
  FastCorr : Scope  Commented=on  NumInputPorts=4
  Golay Correlator 32 : Subsystem  TreatAsAtomicUnit=on
  Logical Operator : Logic  AllPortsSameDT=off  OutDataTypeStr=boolean
  Logical Operator11 : Logic  Inputs=3  AllPortsSameDT=off  OutDataTypeStr=boolean
  Product : Product  OutDataTypeStr=Inherit: Same as first input
  Product1 : Product  OutDataTypeStr=Inherit: Same as first input
  Product2 : Product  OutDataTypeStr=Inherit: Same as first input
  Real-Imag to Complex : RealImagToComplex
  Real-Imag to Complex1 : RealImagToComplex
  Real-Imag to Complex2 : RealImagToComplex
  RxRaisedCosine2 : Subsystem  TreatAsAtomicUnit=on
  Switch : Switch
  Switch1 : Switch  Criteria=u2 > Threshold
  Switch2 : Switch  Criteria=u2 > Threshold
  Terminator : Terminator
  agc_settled : simulink/Logic and Bit Operations/Compare To Constant  relop=<=  const=agcSettleThresh  OutDataTypeStr=boolean
  agc_settled1 : simulink/Logic and Bit Operations/Compare To Constant  relop=>=  const=-agcSettleThresh  OutDataTypeStr=boolean
  average_filter : Subsystem  AncestorBlock=helperLib/average_filter  mask{pipe=regular_pipeline, samples=agcPwrAvgNum, gain=1/agcPwrAvgNum}
      mask prompts: pipe "Pipeline Delay"; samples "Samples to Average Over"; gain "Gain to Multiply Each Sample By"
  complex_magnitude_sq_cfg : helperLib/complex_magnitude_sq_cfg  mult=mult_pipeline  pipe=regular_pipeline
  complex_magnitude_sq_cfg1 : helperLib/complex_magnitude_sq_cfg  mult=mult_pipeline  pipe=regular_pipeline
  pipeline_delay : Delay  DelayLength=regular_pipeline*3
  pipeline_delay{2..7,16..17,20..26} (15 alike) : Delay  DelayLength=regular_pipeline
  pipeline_delay_match : Delay  DelayLength=(regular_pipeline*12+mult_pipeline*3+4)+agc_delay_lag
  pipeline_delay_match1 : Delay  DelayLength=regular_pipeline*7+golay_type
  pipelined_mult : helperLib/pipelined_mult  d=wide_mult_pipeline
  pipelined_mult{1..4} (4 alike) : helperLib/pipelined_mult  d=mult_pipeline
  preamble_detect : Stateflow chart  TreatAsAtomicUnit=on
      settings: RTWSystemCode=Reusable function
  sig_out_i : Outport
  sig_out_q : Outport  Port=2
  rawI : Outport  Port=3
  rawQ : Outport  Port=4
  agcPwrEst : Outport  Port=5
  agcCorrection : Outport  Port=6
  preamble_detected : Outport  Port=7
  preamble_err : Outport  Port=8
  wires:
  agc_on/1 -> pipeline_delay5/1
  Add/1 -> Product1/1
  agc_freeze/1 -> Logical Operator/1
  pipeline_delay16/1 -> AGC/5(agc_sat_up)
  agc_sat_low/1 -> pipeline_delay17/1
  Data Type Conversion/1 -> pipelined_mult/1
  Switch/1 -> agcCorrection/1, Delay12/1
  pipeline_delay4/1 -> Product/2
  gain/1 -> pipeline_delay4/1
  pre_gain_q/1 -> pipeline_delay2/1
  pre_gain_i/1 -> pipeline_delay3/1
  pipeline_delay20/1 -> Add/1
  Logical Operator/1 -> AGC/4(freeze)
  Real-Imag to Complex/1 -> pipeline_delay24/1
  pipeline_delay17/1 -> AGC/6(agc_sat_low)
  Add1/1 -> Product2/1
  agc_sat_up/1 -> pipeline_delay16/1
  pipeline_delay25/1 -> rawI/1
  agc_step_size/1 -> pipeline_delay7/1
  baseband_i/1 -> pipeline_delay20/1
  Product1/1 -> Real-Imag to Complex/1, pipeline_delay25/1
  pipeline_delay23/1 -> Add/2
  baseband_q/1 -> pipeline_delay21/1
  agc_desired/1 -> pipeline_delay6/1
  pipeline_delay6/1 -> AGC/2(Desired)
  pipeline_delay7/1 -> AGC/3(Step)
  Product2/1 -> Real-Imag to Complex/2, pipeline_delay26/1
  AGC/1(Correction) -> Switch/1
  pipeline_delay5/1 -> Switch/2
  pipeline_delay26/1 -> rawQ/1
  Constant/1 -> Switch/3
  AGC/2(LnPwr) -> average_filter/1(In1)
  pipeline_delay/1 -> Data Type Conversion/1
  pipeline_delay21/1 -> Add1/1
  freeze_en_agc/1 -> Logical Operator/2
  offset_q/1 -> pipeline_delay22/1
  pipeline_delay22/1 -> Add1/2
  pipeline_delay24/1 -> Product/1
  Product/1 -> pipeline_delay/1
  Data Type Conversion2/1 -> RxRaisedCosine2/1(In2)
  offset_i/1 -> pipeline_delay23/1
  average_filter/1(Out1) -> pipeline_delay_match1/1, pipeline_delay_match/1
  Complex to Real-Imag/1 -> sig_out_i/1
  Complex to Real-Imag/2 -> sig_out_q/1
  Complex to Real-Imag3/1 -> pipelined_mult3/1
  Golay Correlator 32/2(Cb) -> Complex to Real-Imag3/1
  complex_magnitude_sq_cfg/1 -> Compare To Constant4/1, Compare To Constant6/1, FastCorr/1
  Complex to Real-Imag2/1 -> pipelined_mult1/1
  complex_magnitude_sq_cfg1/1 -> Compare To Constant7/1, Compare To Constant1/1, FastCorr/2
  Golay Correlator 32/1(Ca) -> Complex to Real-Imag2/1
  Real-Imag to Complex2/1 -> complex_magnitude_sq_cfg1/1
  Real-Imag to Complex1/1 -> complex_magnitude_sq_cfg/1
  Data Type Conversion1/1 -> Golay Correlator 32/1(In)
  Complex to Real-Imag3/2 -> pipelined_mult4/1
  pipelined_mult4/1 -> Real-Imag to Complex2/2
  Constant1/1 -> pipelined_mult2/2, pipelined_mult1/2, pipelined_mult4/2, pipelined_mult3/2
  pipelined_mult2/1 -> Real-Imag to Complex1/2
  pipelined_mult1/1 -> Real-Imag to Complex1/1
  Complex to Real-Imag2/2 -> pipelined_mult2/1
  pipelined_mult3/1 -> Real-Imag to Complex2/1
  Switch1/1 -> Terminator/1, FastCorr/3
  Switch2/1 -> FastCorr/4, Logical Operator11/3
  agc_settled1/1 -> Logical Operator11/2
  pipeline_delay_match/1 -> agcPwrEst/1
  agc_settled/1 -> Logical Operator11/1
  Constant2/1 -> preamble_detect/2(rst)
  Logical Operator11/1 -> preamble_detect/1(peak)
  preamble_detect/1(err) -> Delay1/1
  preamble_detect/2(detected) -> Delay2/1
  Delay1/1 -> preamble_err/1
  Delay2/1 -> preamble_detected/1
  pipeline_delay2/1 -> Product2/2
  pipeline_delay3/1 -> Product1/2
  Compare To Constant6/1 -> Switch1/1
  Compare To Constant7/1 -> Switch2/1
  Compare To Constant1/1 -> Switch2/3
  Compare To Constant4/1 -> Switch1/3
  preamble_detect/3(possible) -> Delay3/1
  Delay3/1 -> Switch2/2, Switch1/2
  pipeline_delay_match1/1 -> agc_settled1/1, agc_settled/1
  pipelined_mult/1 -> Data Type Conversion2/1
  RxRaisedCosine2/1(Out2) -> Data Type Conversion3/1
  Data Type Conversion3/1 -> Data Type Conversion1/1, Complex to Real-Imag/1, AGC/1(In)
  Delay12/1 -> pipelined_mult/2

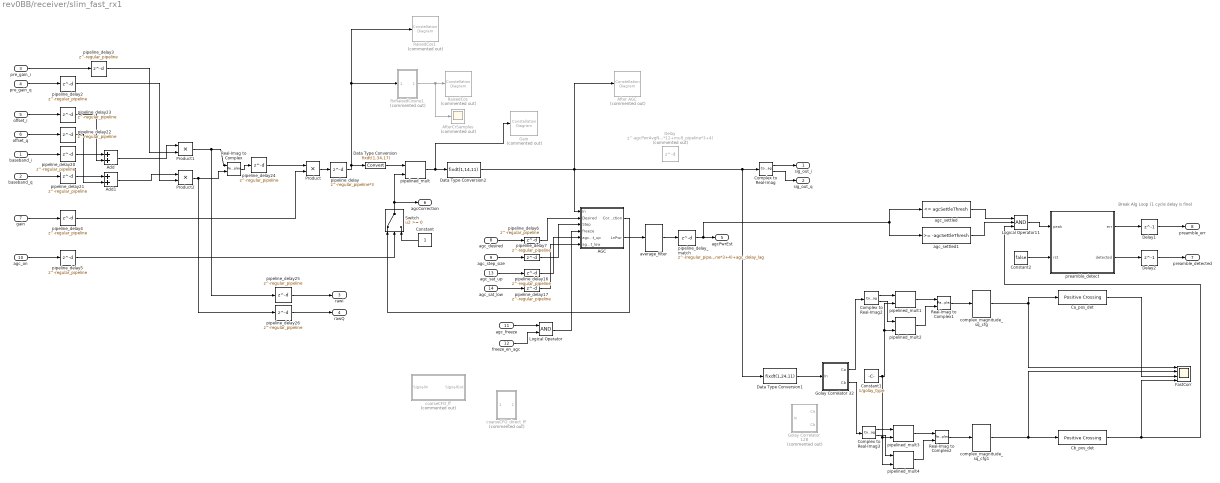
== system rev0BB/receiver/slim_fast_rx1 ==
  note: Break Alg Loop (1 cycle delay is fine)
  baseband_i : Inport
  baseband_q : Inport  Port=2
  pre_gain_i : Inport  Port=3
  pre_gain_q : Inport  Port=4
  offset_i : Inport  Port=5
  offset_q : Inport  Port=6
  gain : Inport  Port=7
  agc_desired : Inport  Port=8
  agc_step_size : Inport  Port=9
  agc_on : Inport  Port=10  OutDataTypeStr=boolean
  agc_freeze : Inport  Port=11  OutDataTypeStr=boolean
  freeze_en_agc : Inport  Port=12  OutDataTypeStr=boolean
  agc_sat_up : Inport  Port=13
  agc_sat_low : Inport  Port=14
  " RaisedCos" : ConstellationDiagram  Commented=on
  " RaisedCos1" : ConstellationDiagram  Commented=on
  AGC : Subsystem
  Add : Sum
  Add1 : Sum
  After AGC : ConstellationDiagram  Commented=on
  AfterCrSamples : Scope  Commented=on
  Ca_pos_det : helperLib/Positive Crossing  crossPt=trigger
  Cb_pos_det : helperLib/Positive Crossing  crossPt=trigger
  Complex to Real-Imag : ComplexToRealImag
  Complex to Real-Imag2 : ComplexToRealImag
  Complex to Real-Imag3 : ComplexToRealImag
  Constant : Constant  OutDataTypeStr=Inherit: Inherit via back propagation  SampleTime=-1
  Constant1 : Constant  Value=1/golay_type  OutDataTypeStr=Inherit: Inherit via back propagation
  Constant2 : Constant  Value=false  SampleTime=-1
  Data Type Conversion : DataTypeConversion  OutDataTypeStr=fixdt(1,34,17)
  Data Type Conversion1 : DataTypeConversion  OutDataTypeStr=fixdt(1,24,11)
  Data Type Conversion2 : DataTypeConversion  OutDataTypeStr=fixdt(1,14,11)
  Delay : Delay  Commented=on  DelayLength=agcPwrAvgNum/2-(regular_pipeline*12+mult_pipeline*3+4)  InitialCondition=0
  Delay1 : Delay  DelayLength=1  InitialCondition=0
  Delay2 : Delay  DelayLength=1  InitialCondition=0
  FastCorr : Scope  NumInputPorts=4
  Gain : ConstellationDiagram  Commented=on
  Golay Correlator 128 : Subsystem  Commented=on
  Golay Correlator 32 : Subsystem
  Logical Operator : Logic  AllPortsSameDT=off  OutDataTypeStr=boolean
  Logical Operator11 : Logic  Inputs=3  AllPortsSameDT=off  OutDataTypeStr=boolean
  Product : Product  OutDataTypeStr=Inherit: Same as first input
  Product1 : Product  OutDataTypeStr=Inherit: Same as first input
  Product2 : Product  OutDataTypeStr=Inherit: Same as first input
  Real-Imag to Complex : RealImagToComplex
  Real-Imag to Complex1 : RealImagToComplex
  Real-Imag to Complex2 : RealImagToComplex
  RxRaisedCosine1 : Subsystem  Commented=on
  Switch : Switch
  agc_settled : simulink/Logic and Bit Operations/Compare To Constant  relop=<=  const=agcSettleThresh  OutDataTypeStr=boolean
  agc_settled1 : simulink/Logic and Bit Operations/Compare To Constant  relop=>=  const=-agcSettleThresh  OutDataTypeStr=boolean
  average_filter : helperLib/average_filter  pipe=regular_pipeline  samples=agcPwrAvgNum  gain=1/agcPwrAvgNum
  coarseCFO_direct_ff : Subsystem  Commented=on
  coarseCFO_ff : Subsystem  Commented=on
  complex_magnitude_sq_cfg : helperLib/complex_magnitude_sq_cfg  mult=mult_pipeline  pipe=regular_pipeline
  complex_magnitude_sq_cfg1 : helperLib/complex_magnitude_sq_cfg  mult=mult_pipeline  pipe=regular_pipeline
  pipeline_delay : Delay  DelayLength=regular_pipeline*3
  pipeline_delay{2..7,16..17,20..26} (15 alike) : Delay  DelayLength=regular_pipeline
  pipeline_delay_match : Delay  DelayLength=(regular_pipeline*12+mult_pipeline*3+4)+agc_delay_lag
  pipelined_mult : helperLib/pipelined_mult  d=wide_mult_pipeline
  pipelined_mult{1..4} (4 alike) : helperLib/pipelined_mult  d=mult_pipeline
  preamble_detect : Stateflow chart  TreatAsAtomicUnit=on
  sig_out_i : Outport
  sig_out_q : Outport  Port=2
  rawI : Outport  Port=3
  rawQ : Outport  Port=4
  agcPwrEst : Outport  Port=5
  agcCorrection : Outport  Port=6
  preamble_detected : Outport  Port=7
  preamble_err : Outport  Port=8
  wires:
  agc_on/1 -> pipeline_delay5/1
  Add/1 -> Product1/1
  agc_freeze/1 -> Logical Operator/1
  pipeline_delay16/1 -> AGC/5(agc_sat_up)
  agc_sat_low/1 -> pipeline_delay17/1
  Data Type Conversion/1 -> pipelined_mult/1
  Switch/1 -> agcCorrection/1, pipelined_mult/2
  pipeline_delay4/1 -> Product/2
  gain/1 -> pipeline_delay4/1
  pre_gain_q/1 -> pipeline_delay2/1
  pre_gain_i/1 -> pipeline_delay3/1
  pipeline_delay20/1 -> Add/1
  Logical Operator/1 -> AGC/4(freeze)
  Real-Imag to Complex/1 -> pipeline_delay24/1
  pipeline_delay17/1 -> AGC/6(agc_sat_low)
  Add1/1 -> Product2/1
  agc_sat_up/1 -> pipeline_delay16/1
  pipeline_delay25/1 -> rawI/1
  agc_step_size/1 -> pipeline_delay7/1
  baseband_i/1 -> pipeline_delay20/1
  Product1/1 -> Real-Imag to Complex/1, pipeline_delay25/1
  pipeline_delay23/1 -> Add/2
  baseband_q/1 -> pipeline_delay21/1
  agc_desired/1 -> pipeline_delay6/1
  pipeline_delay6/1 -> AGC/2(Desired)
  pipeline_delay7/1 -> AGC/3(Step)
  Product2/1 -> Real-Imag to Complex/2, pipeline_delay26/1
  AGC/1(Correction) -> Switch/1
  pipeline_delay5/1 -> Switch/2
  pipeline_delay26/1 -> rawQ/1
  Constant/1 -> Switch/3
  RxRaisedCosine1/1(Out2) -> AfterCrSamples/1, " RaisedCos"/1
  AGC/2(LnPwr) -> average_filter/1
  pipeline_delay/1 -> Data Type Conversion/1, RxRaisedCosine1/1(In2), " RaisedCos1"/1
  pipeline_delay21/1 -> Add1/1
  freeze_en_agc/1 -> Logical Operator/2
  offset_q/1 -> pipeline_delay22/1
  pipeline_delay22/1 -> Add1/2
  pipelined_mult/1 -> Gain/1, Data Type Conversion2/1
  pipeline_delay24/1 -> Product/1
  Product/1 -> pipeline_delay/1
  Data Type Conversion2/1 -> After AGC/1, Data Type Conversion1/1, Complex to Real-Imag/1, AGC/1(In)
  offset_i/1 -> pipeline_delay23/1
  average_filter/1 -> pipeline_delay_match/1
  Complex to Real-Imag/1 -> sig_out_i/1
  Complex to Real-Imag/2 -> sig_out_q/1
  Complex to Real-Imag3/1 -> pipelined_mult3/1
  Golay Correlator 32/2(Cb) -> Complex to Real-Imag3/1
  complex_magnitude_sq_cfg/1 -> FastCorr/1, Ca_pos_det/1
  Complex to Real-Imag2/1 -> pipelined_mult1/1
  complex_magnitude_sq_cfg1/1 -> FastCorr/2, Cb_pos_det/1
  Golay Correlator 32/1(Ca) -> Complex to Real-Imag2/1
  Real-Imag to Complex2/1 -> complex_magnitude_sq_cfg1/1
  Real-Imag to Complex1/1 -> complex_magnitude_sq_cfg/1
  Data Type Conversion1/1 -> Golay Correlator 32/1(In)
  Complex to Real-Imag3/2 -> pipelined_mult4/1
  pipelined_mult4/1 -> Real-Imag to Complex2/2
  Constant1/1 -> pipelined_mult2/2, pipelined_mult1/2, pipelined_mult4/2, pipelined_mult3/2
  pipelined_mult2/1 -> Real-Imag to Complex1/2
  pipelined_mult1/1 -> Real-Imag to Complex1/1
  Complex to Real-Imag2/2 -> pipelined_mult2/1
  pipelined_mult3/1 -> Real-Imag to Complex2/1
  Ca_pos_det/1 -> FastCorr/3
  Cb_pos_det/1 -> Logical Operator11/3, FastCorr/4
  agc_settled1/1 -> Logical Operator11/2
  pipeline_delay_match/1 -> agc_settled/1, agc_settled1/1, agcPwrEst/1
  agc_settled/1 -> Logical Operator11/1
  Constant2/1 -> preamble_detect/2(rst)
  Logical Operator11/1 -> preamble_detect/1(peak)
  preamble_detect/1(err) -> Delay1/1
  preamble_detect/2(detected) -> Delay2/1
  Delay1/1 -> preamble_err/1
  Delay2/1 -> preamble_detected/1
  pipeline_delay2/1 -> Product2/2
  pipeline_delay3/1 -> Product1/2
